simulink model "unicycle_control_Exercise3"  (R2017b)
settings: Solver=ode45  StartTime=0.0  StopTime=100  RelTol=1e-3
InitFcn:
  | parametersUnicycle
StopFcn:
  | outputplotExercise3
values from neighbouring files (symbols this model uses):
  accel_limit = 1    [parametersUnicycle.m]
  b = 0.5    [parametersUnicycle.m]
  drive_limit = 10    [parametersUnicycle.m]
  f = 0.01    [geometricParams.m]
  k1 = 1    [parametersUnicycle.m]
  k2 = 1    [parametersUnicycle.m]
  Pf = [0 4 0]    [geometricParams.m]
  Pi = [0 0 0 ]    [geometricParams.m]
  r = 2    [geometricParams.m]
  steer_limit = 10    [parametersUnicycle.m]
  x0 = Pi    [parametersUnicycle.m]
undefined symbols (not defined in the file or in its folder): angdiff
libraries: simulink x2
settings Model: Creator=jan.rosell  LastModifiedBy=linux
settings DataIOCC: LimitDataPoints=on  SaveFormat=Array  SignalLoggingSaveFormat=ModelDataLogs
settings OptimizationCC: BlockReduction=off  BooleanDataType=off  ExpressionDepthLimit=2147483647  LifeSpan=inf
settings DebuggingCC: SaveWithParameterizedLinksMsg=none  UnderspecifiedInitializationDetection=Classic  MergeDetectMultiDrivingBlocksExec=none  SignalResolutionControl=TryResolveAllWithWarning  MultiTaskDSMMsg=warning  MultiTaskCondExecSysMsg=none  StateNameClashWarn=warning  StrictBusMsg=None  SFUnexpectedBacktrackingDiag=warning  SFNoUnconditionalDefaultTransitionDiag=warning  SFExecutionAtInitializationDiag=none
settings HardwareCC: ProdBitPerPointer=32  ProdBitPerSizeT=32  ProdBitPerPtrDiffT=32  ProdLargestAtomicFloat=None  ProdIntDivRoundTo=Undefined  ProdEndianess=Unspecified  ProdWordSize=32  ProdHWDeviceType=32-bit Generic  TargetUnknown=on
settings ModelReferenceCC: PropagateSignalLabelsOutOfModel=off
settings CodeAppCC: StateflowObjectComments=on
settings GRTTargetCC: TargetLangStandard=C89/C90 (ANSI)  GeneratePreprocessorConditionals=Disable all
settings ConfigComp: CovMetricSettings=dw  CovHtmlReporting=on  CovSaveCumulativeToWorkspaceVar=on  CovSaveSingleToWorkspaceVar=on  CovExternalEMLEnable=off

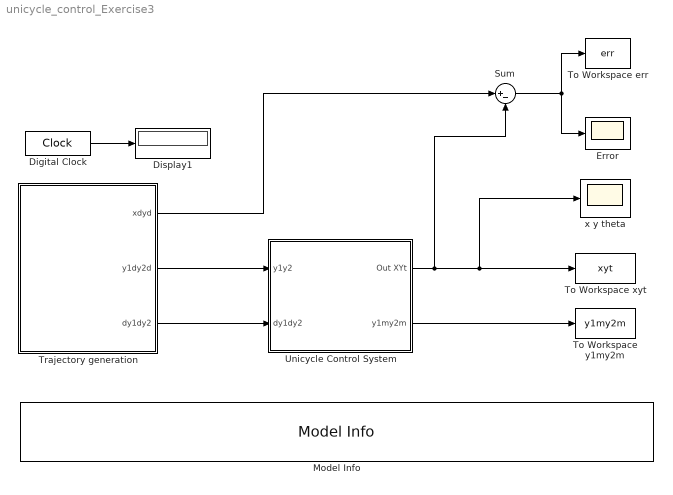
== system unicycle_control_Exercise3 ==
  Digital Clock : DigitalClock
  Display1 : Display
  Error : Scope
  Model Info : simulink/Model-Wide Utilities/Model Info  Frame=on  DisplayStringWithTags=|  HorizontalTextAlignment=Left  LeftAlignmentValue=0.02
      | The file parametersUnicycle.m contain some parameters of the model and is executed upon running the model. 
      | 
      | Modify the values in this file as required.
  Sum : Sum  Inputs=|+-
  To Workspace err : ToWorkspace  VariableName=err  SampleTime=-1
  "To Workspace xyt " : ToWorkspace  VariableName=xyt  SampleTime=-1
  "To Workspace y1my2m " : ToWorkspace  VariableName=y1my2m  SampleTime=-1
  Trajectory generation : Subsystem
  Unicycle Control System : Subsystem
  x y theta : Scope
  wires:
  Unicycle Control System/1(Out XYt) -> "To Workspace xyt "/1, x y theta/1, Sum/2
  Unicycle Control System/2(y1my2m) -> "To Workspace y1my2m "/1
  Sum/1 -> Error/1, To Workspace err/1
  Trajectory generation/1(" xdyd") -> Sum/1
  Trajectory generation/3(" dy1dy2") -> Unicycle Control System/2(dy1dy2)
  Trajectory generation/2(y1dy2d) -> Unicycle Control System/1("y1y2 ")
  Digital Clock/1 -> Display1/1

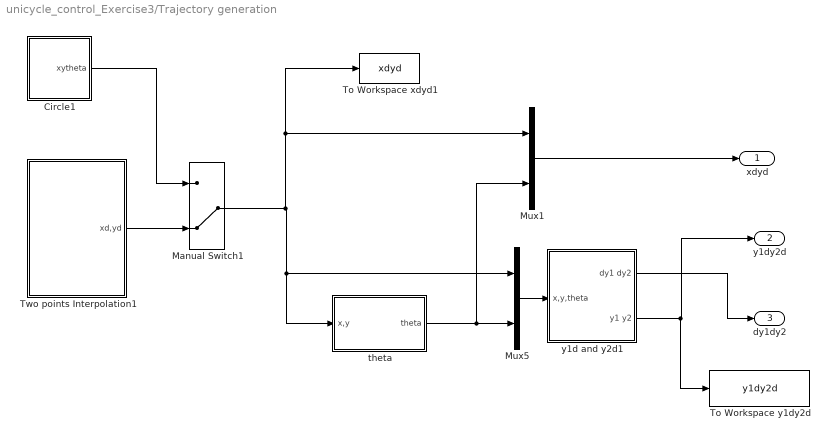
== system unicycle_control_Exercise3/Trajectory generation ==
  Circle1 : Subsystem  mask{radius=r, freq=f}
      mask prompts: freq "Frequency (rev/s)"
      mask help: Generate circular trajectory
      mask Help:
      | Generate circular trajectory in the xy-plane and centred at the origin.
      | 
      | <b>Parameters::</b>
      | 
      | radius   The radius of the circle [m]
      | freq     The frequency of motion [rev/s]
      | 
      | <b>Output::</b>
      | 
      | xy (1x2) a vector of xy-coordinates at the current simulation time step.
      | 
      | <b>Notes::</b>
      | - Motion is at constant velocity around the circle, there is an infinite
      |   initial acceleration.
      | - The motion continues for the whole simulation.
  Manual Switch1 : ManualSwitch  CurrentSetting=0
  Mux1 : Mux  Inputs=2
  Mux5 : Mux  Inputs=2
  To Workspace xdyd1 : ToWorkspace  VariableName=xdyd  SampleTime=-1
  To Workspace y1dy2d : ToWorkspace  VariableName=y1dy2d  SampleTime=-1
  Two points Interpolation1 : Subsystem  mask{Pi=Pi, Pf=Pf, k=10, tmax=100}
      mask prompts: Pi "[xi yi thetai]"; Pf "[xf yf thetaf]"; k "k (interpolation)"; tmax "Duration"
  theta : Subsystem  mask{sense=0}
      mask prompts: sense "0: forward direction; 1: backward direction"
  y1d and y2d1 : Subsystem  mask{b=b}
  " xdyd" : Outport
  y1dy2d : Outport  Port=2
  " dy1dy2" : Outport  Port=3
  wires:
  Mux5/1 -> y1d and y2d1/1(x,y,theta)
  theta/1(theta) -> Mux1/2, Mux5/2
  y1d and y2d1/1(dy1 dy2) -> " dy1dy2"/1
  y1d and y2d1/2(y1 y2) -> To Workspace y1dy2d/1, y1dy2d/1
  Two points Interpolation1/1(xd,yd) -> Manual Switch1/2
  Circle1/1(xytheta) -> Manual Switch1/1
  Manual Switch1/1 -> Mux1/1, To Workspace xdyd1/1, theta/1(x,y), Mux5/1
  Mux1/1 -> " xdyd"/1

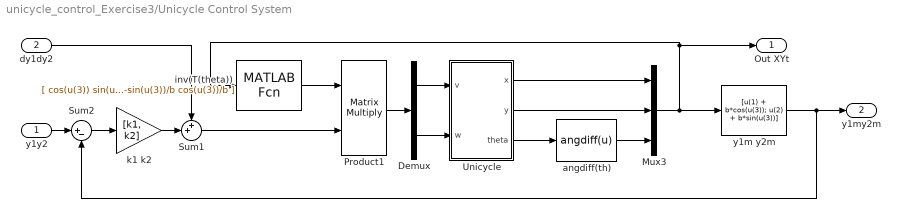
== system unicycle_control_Exercise3/Unicycle Control System ==
  "y1y2 " : Inport
  dy1dy2 : Inport  Port=2
  Demux : Demux  Outputs=2
  Mux3 : Mux  Inputs=3
  Product1 : Product  Multiplication=Matrix(*)  RndMeth=Zero
  Sum1 : Sum  Inputs=++|
  Sum2 : Sum  Inputs=|+-
  "Unicycle " : Subsystem  mask{accel=accel_limit, vdlim=drive_limit, vslim=steer_limit, x0=x0, handbrake=0}
      mask prompts: accel "Acceleration"; vdlim "Drive limit"; vslim "Steering limits"; x0 "Initial state (x, y, theta)"
      mask help: Kino-dynamic model of bicycle vehicle - Siciliano
      mask Help:
      | Kino-dynamic model of bicycle vehicle, also known as Ackermann vehicle
      | model.
      | 
      | <b>Parameters::</b>
      | 
      | Acceleration (1x1)   Vehicle acceleration limit [m/s2]
      | Velocity limit (1x1)  Vehicle speed limit [m/s]
      | Steering limits (1x1) Steering angle limit [rad]
      | Initial state (1x3) Initial state (x, y, theta)
      | Handbrake (1x1) Vehicle cannot move if non-zero
      | 
      | <b>Inputs::</b>
      | 
      | v (1x1) velocity demand [m/s]
      | gamma (1x1) steering angle [rad]
      | 
      | <b>Outputs::</b>
      | 
      | x (1x1) x-coordinate in world frame [m]
      | y (1x1) x-coordinate in world frame [m]
      | theta (1x1) heading angle in world frame [rad]
      | 
      | 
      | <b>Notes::</b>
      | 
      | - Steering limit is symmetric between -limit and +limit
      | - Same dynamic model as the Toolbox class Vehicle.
  angdiff(th) : MATLABFcn  MATLABFcn=angdiff(u)
  "inv(T(theta)) " : MATLABFcn  MATLABFcn=[ cos(u(3)) sin(u(3)); -sin(u(3))/b cos(u(3))/b ]  OutputDimensions=[2 2]  Output1D=off
  k1 k2 : Gain  Gain=[k1, k2]
  y1m y2m : MATLABFcn  MATLABFcn=[u(1) + b*cos(u(3)); u(2) + b*sin(u(3))]  OutputDimensions=[2]  Output1D=off
  Out XYt : Outport
  y1my2m : Outport  Port=2
  wires:
  k1 k2/1 -> Sum1/2
  Sum1/1 -> Product1/2
  "Unicycle "/2(y) -> Mux3/2
  "Unicycle "/3(theta) -> angdiff(th)/1
  Mux3/1 -> Out XYt/1, "inv(T(theta)) "/1, y1m y2m/1
  y1m y2m/1 -> Sum2/2, y1my2m/1
  "inv(T(theta)) "/1 -> Product1/1
  Product1/1 -> Demux/1
  Demux/1 -> "Unicycle "/1(v)
  Demux/2 -> "Unicycle "/2(w)
  Sum2/1 -> k1 k2/1
  "Unicycle "/1(x) -> Mux3/1
  angdiff(th)/1 -> Mux3/3
  "y1y2 "/1 -> Sum2/1
  dy1dy2/1 -> Sum1/1

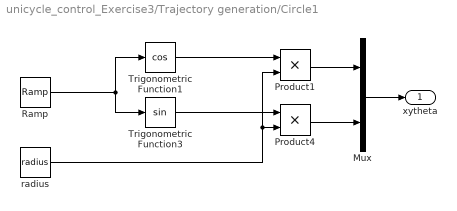
== system unicycle_control_Exercise3/Trajectory generation/Circle1 ==
  Mux : Mux  Inputs=2
  Product1 : Product  RndMeth=Zero
  Product4 : Product  RndMeth=Zero
  Ramp : simulink/Sources/Ramp  slope=freq*2*pi  start=0  X0=0
  Trigonometric Function1 : Trigonometry  Operator=cos
  Trigonometric Function3 : Trigonometry
  radius : Constant  Value=radius
  xytheta : Outport
  wires:
  radius/1 -> Product1/2, Product4/2
  Mux/1 -> xytheta/1
  Ramp/1 -> Trigonometric Function3/1, Trigonometric Function1/1
  Trigonometric Function3/1 -> Product4/1
  Trigonometric Function1/1 -> Product1/1
  Product1/1 -> Mux/1
  Product4/1 -> Mux/2

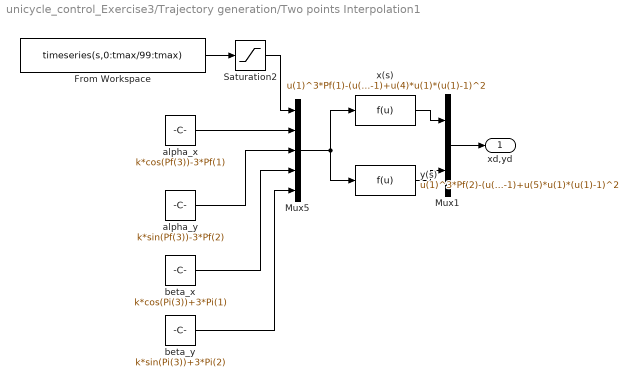
== system unicycle_control_Exercise3/Trajectory generation/Two points Interpolation1 ==
  From Workspace : FromWorkspace  VariableName=timeseries(s,0:tmax/99:tmax)  SampleTime=0
  Mux1 : Mux  Inputs=2
  Mux5 : Mux  Inputs=5
  Saturation2 : Saturate  UpperLimit=1  LowerLimit=0
  alpha_x : Constant  Value=k*cos(Pf(3))-3*Pf(1)
  alpha_y : Constant  Value=k*sin(Pf(3))-3*Pf(2)
  beta_x : Constant  Value=k*cos(Pi(3))+3*Pi(1)
  beta_y : Constant  Value=k*sin(Pi(3))+3*Pi(2)
  x(s) : Fcn  Expr=u(1)^3*Pf(1)-(u(1)-1)^3*Pi(1)+u(2)*u(1)^2*(u(1)-1)+u(4)*u(1)*(u(1)-1)^2
  y(s) : Fcn  Expr=u(1)^3*Pf(2)-(u(1)-1)^3*Pi(2)+u(3)*u(1)^2*(u(1)-1)+u(5)*u(1)*(u(1)-1)^2
  xd,yd : Outport
  wires:
  alpha_x/1 -> Mux5/2
  alpha_y/1 -> Mux5/3
  beta_x/1 -> Mux5/4
  beta_y/1 -> Mux5/5
  Mux5/1 -> x(s)/1, y(s)/1
  From Workspace/1 -> Saturation2/1
  Saturation2/1 -> Mux5/1
  x(s)/1 -> Mux1/1
  y(s)/1 -> Mux1/2
  Mux1/1 -> xd,yd/1

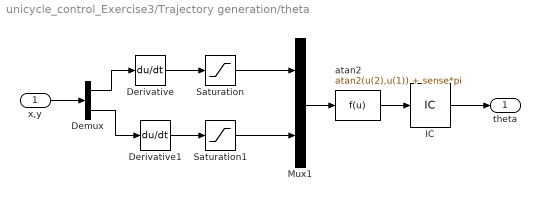
== system unicycle_control_Exercise3/Trajectory generation/theta ==
  x,y : Inport
  Demux : Demux  Outputs=2
  Derivative : Derivative  CoefficientInTFapproximation=100
  Derivative1 : Derivative  CoefficientInTFapproximation=100
  IC : InitialCondition  Value=Pi(3)
  Mux1 : Mux  Inputs=2
  Saturation : Saturate  UpperLimit=1  LowerLimit=-1  ZeroCross=off
  Saturation1 : Saturate  UpperLimit=1  LowerLimit=-1  ZeroCross=off
  atan2 : Fcn  Expr=atan2(u(2),u(1)) + sense*pi
  theta : Outport
  wires:
  Mux1/1 -> atan2/1
  Saturation/1 -> Mux1/1
  Derivative1/1 -> Saturation1/1
  Derivative/1 -> Saturation/1
  Saturation1/1 -> Mux1/2
  IC/1 -> theta/1
  atan2/1 -> IC/1
  Demux/1 -> Derivative/1
  Demux/2 -> Derivative1/1
  x,y/1 -> Demux/1

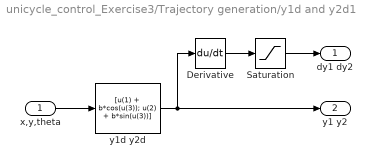
== system unicycle_control_Exercise3/Trajectory generation/y1d and y2d1 ==
  x,y,theta : Inport
  Derivative : Derivative  CoefficientInTFapproximation=100
  Saturation : Saturate  UpperLimit=1  LowerLimit=-1  ZeroCross=off
  y1d y2d : MATLABFcn  MATLABFcn=[u(1) + b*cos(u(3)); u(2) + b*sin(u(3))]  OutputDimensions=[2]  Output1D=off
  dy1 dy2 : Outport
  y1 y2 : Outport  Port=2
  wires:
  x,y,theta/1 -> y1d y2d/1
  y1d y2d/1 -> y1 y2/1, Derivative/1
  Derivative/1 -> Saturation/1
  Saturation/1 -> dy1 dy2/1

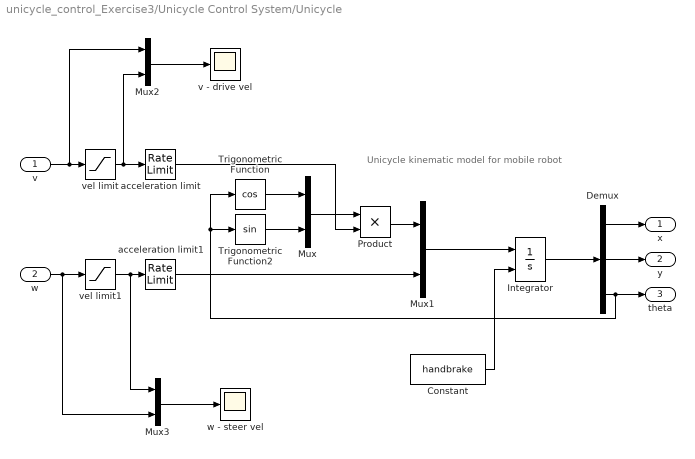
== system unicycle_control_Exercise3/Unicycle Control System/Unicycle  ==
  note: Unicycle kinematic model for mobile robot
  v : Inport
  w : Inport  Port=2
  Constant : Constant  Value=handbrake
  Demux : Demux  Outputs=3
  Integrator : Integrator  ExternalReset=level  InitialCondition=x0
  Mux{,1..3} (4 alike) : Mux  Inputs=2
  Product : Product  RndMeth=Zero
  Trigonometric Function : Trigonometry  Operator=cos
  Trigonometric Function2 : Trigonometry
  acceleration limit : RateLimiter  RisingSlewLimit=accel  FallingSlewLimit=-accel
  acceleration limit1 : RateLimiter  RisingSlewLimit=accel*100  FallingSlewLimit=-accel*100
  v - drive vel : Scope
  vel limit : Saturate  UpperLimit=vdlim  LowerLimit=-vdlim  ZeroCross=off
  vel limit1 : Saturate  UpperLimit=vslim  LowerLimit=-vslim  ZeroCross=off
  w - steer vel : Scope
  x : Outport
  y : Outport  Port=2
  theta : Outport  Port=3
  wires:
  Trigonometric Function/1 -> Mux/1
  acceleration limit/1 -> Product/2
  Integrator/1 -> Demux/1
  Demux/3 -> Trigonometric Function/1, Trigonometric Function2/1, theta/1
  Demux/1 -> x/1
  Demux/2 -> y/1
  Mux/1 -> Product/1
  Trigonometric Function2/1 -> Mux/2
  Constant/1 -> Integrator/2
  w/1 -> Mux3/2, vel limit1/1
  Product/1 -> Mux1/1
  acceleration limit1/1 -> Mux1/2
  Mux1/1 -> Integrator/1
  vel limit1/1 -> Mux3/1, acceleration limit1/1
  v/1 -> Mux2/1, vel limit/1
  Mux2/1 -> v - drive vel/1
  vel limit/1 -> Mux2/2, acceleration limit/1
  Mux3/1 -> w - steer vel/1
